simulink model "input_value"  (R2015b)
settings: Solver=VariableStepAuto  StartTime=0.0  StopTime=10.0  RelTol=1e-3
settings Model: Creator=yuji  LastModifiedBy=yuji

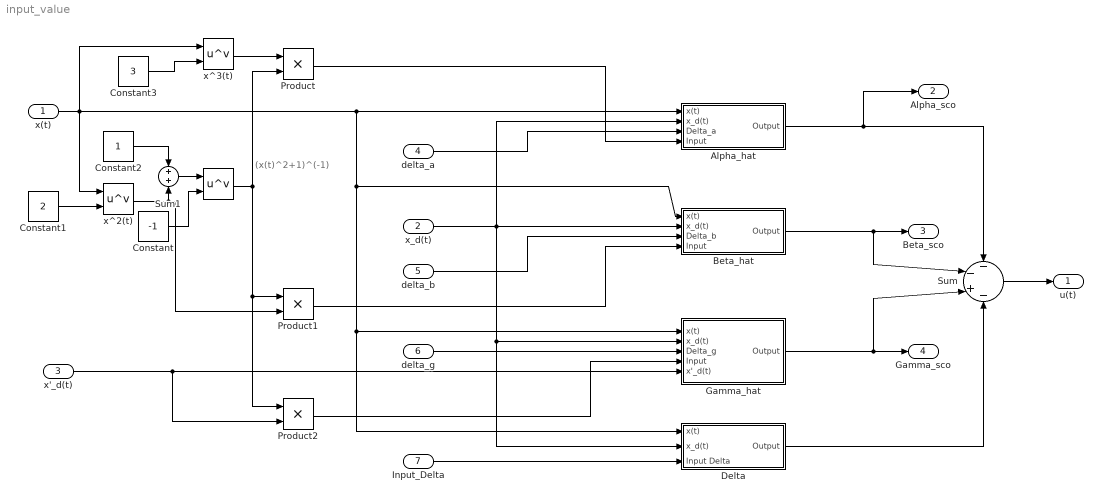
== system input_value ==
  note: (x(t)^2+1)^(-1)
  x(t) : Inport
  x_d(t) : Inport  Port=2
  x'_d(t) : Inport  Port=3
  delta_a : Inport  Port=4
  delta_b : Inport  Port=5
  delta_g : Inport  Port=6
  Input_Delta : Inport  Port=7
  " " : Math  Operator=pow  SaturateOnIntegerOverflow=on
  " x^2(t)" : Math  Operator=pow  SaturateOnIntegerOverflow=on
  " x^3(t)" : Math  Operator=pow  SaturateOnIntegerOverflow=on
  Alpha_hat : Subsystem
  Beta_hat : Subsystem
  Constant : Constant  Value=-1
  Constant1 : Constant  Value=2
  Constant2 : Constant
  Constant3 : Constant  Value=3
  Delta : Subsystem
  Gamma_hat : Subsystem
  Product : Product
  Product1 : Product
  Product2 : Product
  Sum : Sum  Inputs=--+-
  Sum1 : Sum  Inputs=+|+
  u(t) : Outport
  Alpha_sco : Outport  Port=2
  Beta_sco : Outport  Port=3
  Gamma_sco : Outport  Port=4
  wires:
  Sum/1 -> u(t)/1
  Delta/1("Output ") -> Sum/4
  Gamma_hat/1(Output) -> Gamma_sco/1, Sum/3
  Beta_hat/1(Output) -> Beta_sco/1, Sum/2
  Alpha_hat/1(Output) -> Alpha_sco/1, Sum/1
  x(t)/1 -> Alpha_hat/1(x(t)), Delta/1(x(t)), Gamma_hat/1(x(t)), Beta_hat/1(x(t)), " x^3(t)"/1, " x^2(t)"/1
  x_d(t)/1 -> Gamma_hat/2(x_d(t)), Delta/2(x_d(t)), Beta_hat/2(x_d(t)), Alpha_hat/2(x_d(t))
  delta_a/1 -> Alpha_hat/3(Delta_a)
  delta_b/1 -> Beta_hat/3(Delta_b)
  delta_g/1 -> Gamma_hat/3(Delta_g)
  x'_d(t)/1 -> Product2/2, Gamma_hat/5(x'_d(t))
  Input_Delta/1 -> Delta/3(Input Delta)
  Constant/1 -> " "/2
  Constant1/1 -> " x^2(t)"/2
  Constant2/1 -> Sum1/1
  Sum1/1 -> " "/1
  Constant3/1 -> " x^3(t)"/2
  " x^3(t)"/1 -> Product/1
  " "/1 -> Product/2, Product2/1, Product1/1
  Product/1 -> Alpha_hat/4(Input)
  Product1/1 -> Beta_hat/4(Input)
  Product2/1 -> Gamma_hat/4(Input)
  " x^2(t)"/1 -> Product1/2, Sum1/2

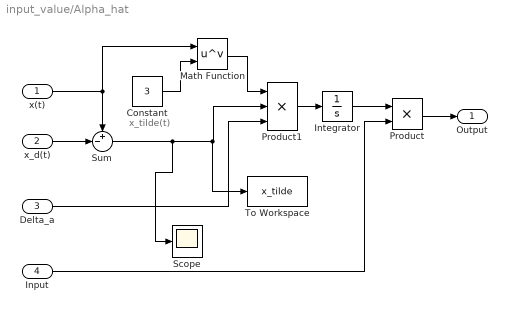
== system input_value/Alpha_hat ==
  note: x_tilde(t)
  x(t) : Inport
  x_d(t) : Inport  Port=2
  Delta_a : Inport  Port=3
  Input : Inport  Port=4
  Constant : Constant  Value=3
  Integrator : Integrator
  Math Function : Math  Operator=pow  SaturateOnIntegerOverflow=on
  Product : Product
  Product1 : Product  Inputs=3
  Scope : Scope
  Sum : Sum  Inputs=+-|
  To Workspace : ToWorkspace  VariableName=x_tilde  SaveFormat=Timeseries  SampleTime=-1
  Output : Outport
  wires:
  Product/1 -> Output/1
  Input/1 -> Product/2
  Integrator/1 -> Product/1
  Product1/1 -> Integrator/1
  Delta_a/1 -> Product1/3
  x_d(t)/1 -> Sum/2
  Sum/1 -> To Workspace/1, Product1/2, Scope/1
  x(t)/1 -> Sum/1, Math Function/1
  Constant/1 -> Math Function/2
  Math Function/1 -> Product1/1

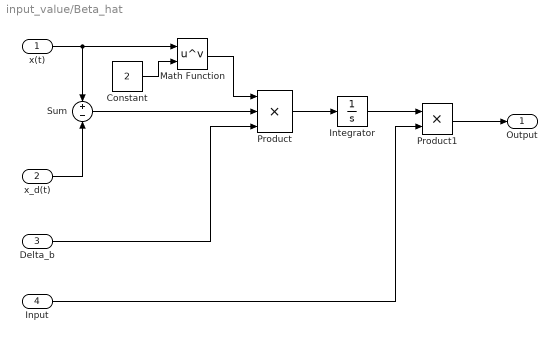
== system input_value/Beta_hat ==
  x(t) : Inport
  x_d(t) : Inport  Port=2
  Delta_b : Inport  Port=3
  Input : Inport  Port=4
  Constant : Constant  Value=2
  Integrator : Integrator
  Math Function : Math  Operator=pow  SaturateOnIntegerOverflow=on
  Product : Product  Inputs=3
  Product1 : Product
  Sum : Sum  Inputs=+|-
  Output : Outport
  wires:
  x(t)/1 -> Math Function/1, Sum/1
  x_d(t)/1 -> Sum/2
  Sum/1 -> Product/2
  Delta_b/1 -> Product/3
  Product/1 -> Integrator/1
  Integrator/1 -> Product1/1
  Product1/1 -> Output/1
  Input/1 -> Product1/2
  Constant/1 -> Math Function/2
  Math Function/1 -> Product/1

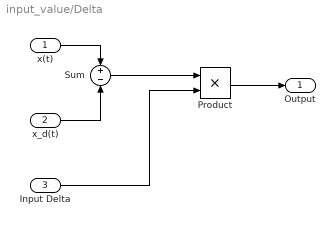
== system input_value/Delta ==
  x(t) : Inport
  x_d(t) : Inport  Port=2
  Input Delta : Inport  Port=3
  Product : Product
  Sum : Sum  Inputs=+|-
  "Output " : Outport
  wires:
  x(t)/1 -> Sum/1
  x_d(t)/1 -> Sum/2
  Sum/1 -> Product/1
  Product/1 -> "Output "/1
  Input Delta/1 -> Product/2

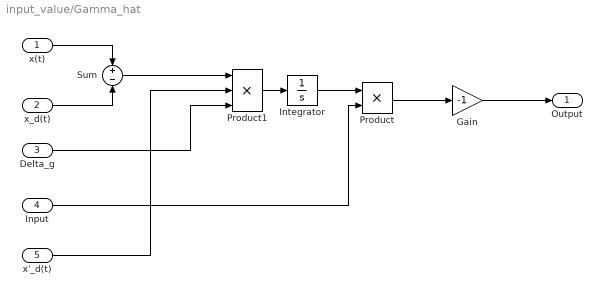
== system input_value/Gamma_hat ==
  x(t) : Inport
  x_d(t) : Inport  Port=2
  Delta_g : Inport  Port=3
  Input : Inport  Port=4
  x'_d(t) : Inport  Port=5
  Gain : Gain  Gain=-1
  Integrator : Integrator
  Product : Product
  Product1 : Product  Inputs=3
  Sum : Sum  Inputs=+|-
  Output : Outport
  wires:
  x(t)/1 -> Sum/1
  x_d(t)/1 -> Sum/2
  Integrator/1 -> Product/1
  Input/1 -> Product/2
  Product1/1 -> Integrator/1
  Sum/1 -> Product1/1
  Delta_g/1 -> Product1/3
  Product/1 -> Gain/1
  Gain/1 -> Output/1
  x'_d(t)/1 -> Product1/2
